simulink library "custom_blocks"  (R2019b)
settings: Solver=VariableStepAuto  StartTime=0.0  StopTime=10.0  RelTol=1e-3
undefined symbols (not defined in the file): aMode, National_Instruments, PCIe, samp
libraries: simulink x25, powerlib_meascontrol x9, $bdroot x2, sldrtlib x1
(part 1 of 2)
settings Model: Creator=guy-m  LastModifiedBy=guy-m

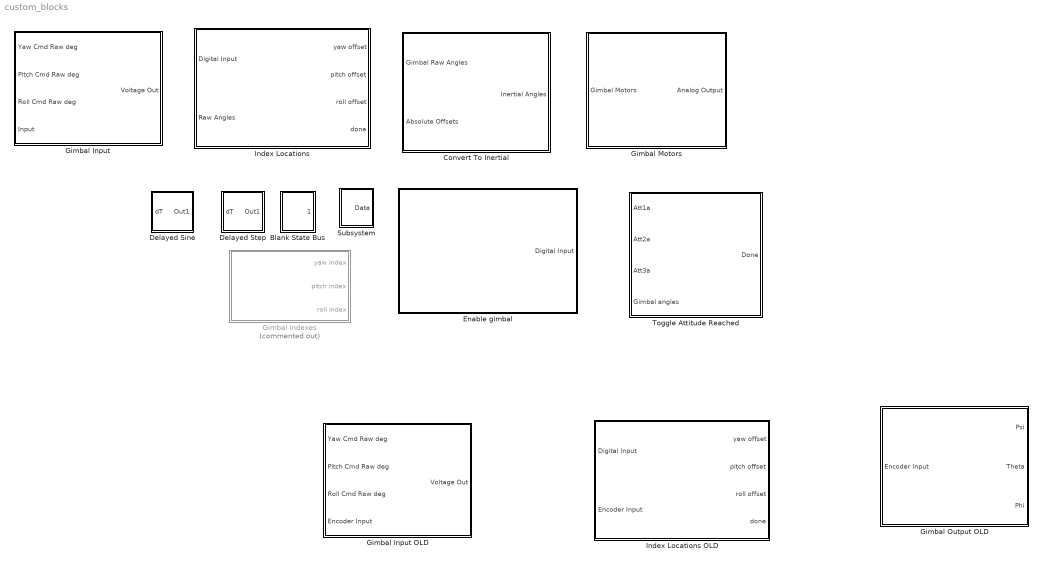
== system custom_blocks ==
  Blank State Bus : Subsystem
      mask DialogControl DescTextVar Prompt: Just a sample state bus object
      mask Display: disp("Blank\nState\nBus")
  Convert To Inertial : Subsystem
      mask init:
      | requiredBlock = find_system(bdroot,'name','Enable gimbal');
      | yawOffset = str2num(get_param(requiredBlock{1},'yawOffset'));
      | pitchOffset = str2num(get_param(requiredBlock{1},'pitchOffset'));
      | rollOffset = str2num(get_param(requiredBlock{1},'rollOffset'));
      mask Display:
      | text(0.5,1," Raw 2 Inertial \n (degrees)",'verticalAlignment','top',"horizontalAlignment",'center')
      | port_label('output',1,'Inertial Angles','texmode','on');
      | port_label('input',1,'Raw Output','texmode','on');
      | port_label('input',2,'Abs. Offsets','texmode','on');
  Delayed Sine : Subsystem  mask{amp=1, bias=5, freq=pi, phase=pi, onTime=0, duration=inf}
      mask DialogControl Control2 Prompt: Amplitude:
      mask DialogControl Control3 Prompt: Bias:
      mask DialogControl Control4 Prompt: Frequency (rad/s):
      mask DialogControl Control5 Prompt: Phase (rad):
      mask DialogControl Control6_copy Prompt: Relative On-Time (s)
      mask DialogControl Control6 Prompt: Duration (s)
      mask Display:
      | port_label('output',1,'','texmode','off');
      | port_label('input',1,'dt','texmode','on');
      | 
      | x = 0:0.001:1;
      | y = sin(2*pi*x);
      | 
      | x = [0,(x+0.5)];
      | y = [0,y];
      | 
      | plot(x,y)
  Delayed Step : Subsystem  mask{stepTime=1, u0=5, u1=pi}
      mask help: This block is similar to a step input, except that the step time is delayed by the block input value (in seconds)
      mask DialogControl Control2 Prompt: Step time:
      mask DialogControl Control3 Prompt: Initial value:
      mask DialogControl Control4 Prompt: Final value:
      mask Display:
      | port_label('output',1,'','texmode','off');
      | port_label('input',1,'dt','texmode','on');
      | if u1>=u0
      |     x = [0.1 0.5 0.5 0.9];
      |     y = [0.1 0.1 0.9 0.9];
      | else
      |     x = [0.1 0.5 0.5 0.9];
      |     y = [0.9 0.9 0.1 0.1];
      | end
      | 
      | plot(x,y)
  Enable gimbal : Subsystem  mask{yawOffset=0, pitchOffset=0, rollOffset=0}
      mask DialogControl DescTextVar Prompt: This block is required in order to enable interfacing with the flight table
      mask DialogControl Control2 Prompt: Yaw Euler Offset
      mask DialogControl Control3 Prompt: Pitch Euler Offset
      mask DialogControl Control4 Prompt: Roll Euler Offset
      mask Display:
      | text(0.5,1,"Enable Gimbals",'verticalAlignment','top',"horizontalAlignment",'center')
      | 
      | port_label('output',1,'Digital Input','texmode','on');
  Gimbal Indexes : Subsystem  Commented=on
      mask Display:
      | disp("Detect Change\nGimbal Index")
      | port_label('output',1,'Yaw','texmode','on');
      | port_label('output',2,'Pitch','texmode','on');
      | port_label('output',3,'Roll','texmode','on');
  Gimbal Input : Subsystem
      mask init: same as custom_blocks/Convert To Inertial
      mask DialogControl DescTextVar Prompt: This block send the raw attitude angles to the gimbal
      mask Display:
      | disp("Gimbal Input\n(degrees)");
      | port_label('input',1,'Yaw','texmode','on');
      | port_label('input',2,'Pitch','texmode','on');
      | port_label('input',3,'Roll','texmode','on');
      | port_label('input',4,'Input','texmode','on');
      | port_label('output',1,'Motors','texmode','on');
  Gimbal Input OLD : Subsystem
      mask init: same as custom_blocks/Convert To Inertial
      mask DialogControl DescTextVar Prompt: This block send the raw attitude angles to the gimbal
      mask Display:
      | disp("Gimbal Input\n(degrees)");
      | port_label('input',1,'Yaw','texmode','on');
      | port_label('input',2,'Pitch','texmode','on');
      | port_label('input',3,'Roll','texmode','on');
      | port_label('input',4,'Encoder Input','texmode','on');
      | port_label('output',1,'Motors','texmode','on');
  Gimbal Motors : Subsystem
      mask DialogControl DescTextVar Prompt: This block controls the DC motors of the gimbal
      mask DialogControl DescTextVar_copy Prompt: A bus object with voltages for each yaw, pitch, and roll motors
      mask Display:
      | text(0.5,1,"Gimbal Motors",'verticalAlignment','top',"horizontalAlignment",'center')
      | 
      | port_label('output',1,"Analog Output",'texmode','on');
      | port_label('input',1,"Motor Voltages",'texmode','on');
  Gimbal Output OLD : Subsystem
      mask init: same as custom_blocks/Convert To Inertial
      mask Display:
      | text(0.5,1," Gimbal Attitude\n (degrees)",'verticalAlignment','top',"horizontalAlignment",'center')
      | port_label('output',1,'Yaw','texmode','on');
      | port_label('output',2,'Pitch','texmode','on');
      | port_label('output',3,'Roll','texmode','on');
      | port_label('input',1,'Encoder Input','texmode','on');
  Index Locations : Subsystem
      mask init: same as custom_blocks/Convert To Inertial
      mask DialogControl DescTextVar Prompt: This block sends (relative) angles at which the physical indexes are found
      mask Display:
      | disp("Gimbal Indexes\n(degrees)")
      | port_label('output',1,'Yaw','texmode','on');
      | port_label('output',2,'Pitch','texmode','on');
      | port_label('output',3,'Roll','texmode','on');
      | port_label('output',4,'Done','texmode','on');
      | port_label('input',1,'Digital Input','texmode','on');
      | port_label('input',2,'Raw Output','texmode','on');
  Index Locations OLD : Subsystem
      mask DialogControl DescTextVar Prompt: This block sends (relative) angles at which the physical indexes are found
      mask Display:
      | disp("Gimbal Indexes\n(degrees)")
      | port_label('output',1,'Yaw','texmode','on');
      | port_label('output',2,'Pitch','texmode','on');
      | port_label('output',3,'Roll','texmode','on');
      | port_label('output',4,'Done','texmode','on');
      | port_label('input',1,'Digital Input','texmode','on');
      | port_label('input',2,'Encoder Input','texmode','on');
  Subsystem : Subsystem
      mask DialogControl ParameterGroupVar Prompt: Just a sample Pixhawk serial message
      mask Display: disp("Blank\nPixhawk\nInput")
  Toggle Attitude Reached : Subsystem
      mask DialogControl DescTextVar Prompt: This block outputs 'true' as soon as both sets of attitude angles coinside. This is a one-time toggle! once turned on, it will remain this way forever.
      mask Display:
      | disp("Toggle Attitude Reached")
      | 
      | port_label('input',1,'Yaw_1','texmode','on');
      | port_label('input',2,'Pitch_1','texmode','on');
      | port_label('input',3,'Roll_1','texmode','on');
      | port_label('input',4,'Encoder Input','texmode','on');
      | port_label('output',1,'Toggle','texmode','on');

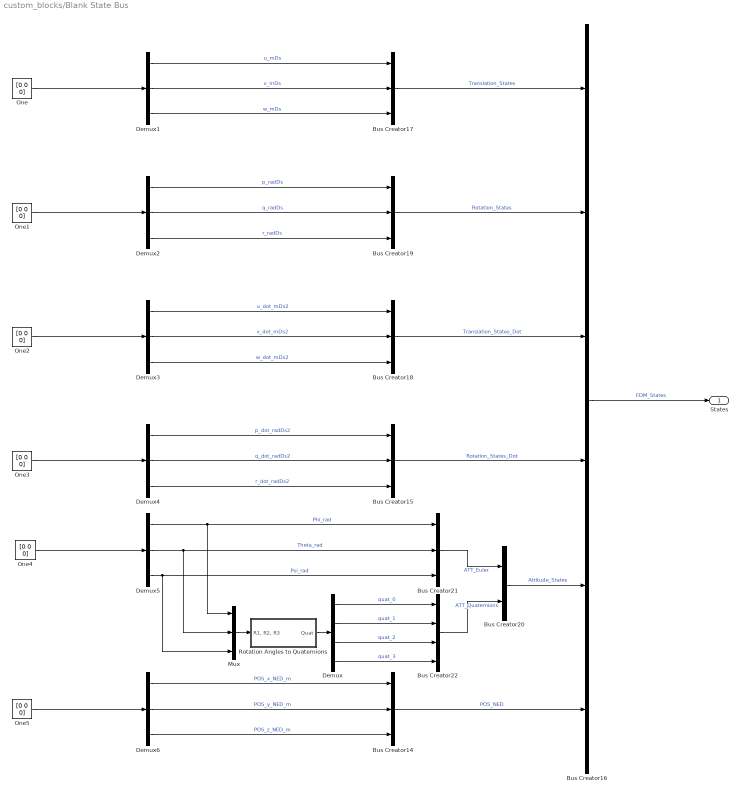
== system custom_blocks/Blank State Bus ==
  Bus Creator{14..15,17..19,21} (6 alike) : BusCreator  Inputs=3
  Bus Creator16 : BusCreator  Inputs=6
  Bus Creator20 : BusCreator  Inputs=2
  Bus Creator22 : BusCreator  Inputs=4
  Demux : Demux
  Demux{1..6} (6 alike) : Demux  Outputs=3
  Mux : Mux  Inputs=3
  One{,1..5} (6 alike) : Constant  Value=[0 0 0]  OutDataTypeStr=Inherit: Inherit via back propagation
  Rotation Angles to Quaternions : Subsystem  mask(Ang2Quat){rotationOrder=ZYX, aMode=aMode}
      mask prompts: rotationOrder "shared_aeroblks:sharedaeroblktransform:blockAng2QuatParamRotationOrder"
      mask help: shared_aeroblks:sharedaeroblktransform:blockAng2QuatDesc
      mask init:
      | if aerosharedtest(gcb)
      |     ports=aerosharedicon('sharedang2quat');
      | else
      |     ports=sharedautoicon('sharedang2quat');
      | end
      settings: AttributesFormatString=Rotation Order: %<rotationOrder>
      mask Help: eval('if license(''test'',''Aerospace_Blockset'')aerosharedhelp(''rotation_angles_to_quaternions'');elseif license(''test'',''Powertrain_Blockset'')sharedautohelp(''rotation_angles_to_quaternions'');end')
      mask TypeOptions rotationOrder: shared_aeroblks:sharedaeroblktransform:blockParamComboZYX | shared_aeroblks:sharedaeroblktransform:blockParamComboZYZ | shared_aeroblks:sharedaeroblktransform:blockParamComboZXY | shared_aeroblks:sharedaeroblktransform:blockParamComboZXZ | shared_aeroblks:sharedaeroblktransform:blockParamComboYXZ | shared_aeroblks:sharedaeroblktransform:blockParamComboYXY | shared_aeroblks:sharedaeroblktransform:blockParamComboYZX | shared_aeroblks:sharedaeroblktransform:blockParamComboYZY | shared_aeroblks:sharedaeroblktransform:blockParamComboXYZ | shared_aeroblks:sharedaeroblktransform:blockParamComboXYX | shared_aeroblks:sharedaeroblktransform:blockParamComboXZY | shared_aeroblks:sharedaeroblktransform:blockParamComboXZX
      mask DialogControl rotationOrder Prompt: Rotation order:
      mask Display:
      | port_label('input',1,'[R_1,R_2,R_3]','texmode','on')
      | port_label('output',1,'q','texmode','on')
  "States " : Outport  VectorParamsAs1DForOutWhenUnconnected=off
  wires:
  One2/1 -> Demux3/1
  Bus Creator22/1 -> Bus Creator20/2  "ATT_Quaternions"
  Bus Creator15/1 -> Bus Creator16/4  "Rotation_States_Dot"
  Demux4/1 -> Bus Creator15/1  "p_dot_radDs2"
  Bus Creator14/1 -> Bus Creator16/6  "POS_NED"
  Demux/3 -> Bus Creator22/3  "quat_2"
  Bus Creator16/1 -> "States "/1  "FDM_States"
  Rotation Angles to Quaternions/1(Quat) -> Demux/1
  Demux/2 -> Bus Creator22/2  "quat_1"
  Demux/4 -> Bus Creator22/4  "quat_3"
  Demux2/2 -> Bus Creator19/2  "q_radDs"
  Mux/1 -> Rotation Angles to Quaternions/1("R1, R2, R3")
  Bus Creator18/1 -> Bus Creator16/3  "Translation_States_Dot"
  Bus Creator17/1 -> Bus Creator16/1  "Translation_States"
  Demux6/1 -> Bus Creator14/1  "POS_x_NED_m"
  Bus Creator21/1 -> Bus Creator20/1  "ATT_Euler"
  Demux6/3 -> Bus Creator14/3  "POS_z_NED_m"
  Bus Creator20/1 -> Bus Creator16/5  "Attitude_States"
  Demux5/2 -> Mux/2, Bus Creator21/2  "Theta_rad"
  Demux5/3 -> Mux/3, Bus Creator21/3  "Psi_rad"
  One1/1 -> Demux2/1
  Demux3/2 -> Bus Creator18/2  "v_dot_mDs2"
  Demux1/2 -> Bus Creator17/2  "v_mDs"
  Demux4/3 -> Bus Creator15/3  "r_dot_radDs2"
  Bus Creator19/1 -> Bus Creator16/2  "Rotation_States"
  Demux2/3 -> Bus Creator19/3  "r_radDs"
  Demux1/1 -> Bus Creator17/1  "u_mDs"
  Demux2/1 -> Bus Creator19/1  "p_radDs"
  Demux3/3 -> Bus Creator18/3  "w_dot_mDs2"
  Demux/1 -> Bus Creator22/1  "quat_0"
  Demux5/1 -> Mux/1, Bus Creator21/1  "Phi_rad"
  Demux1/3 -> Bus Creator17/3  "w_mDs"
  Demux4/2 -> Bus Creator15/2  "q_dot_radDs2"
  Demux6/2 -> Bus Creator14/2  "POS_y_NED_m"
  Demux3/1 -> Bus Creator18/1  "u_dot_mDs2"
  One3/1 -> Demux4/1
  One4/1 -> Demux5/1
  One/1 -> Demux1/1
  One5/1 -> Demux6/1

== system custom_blocks/Convert To Inertial ==
  Gimbal Raw Angles : Inport
  Absolute Offsets : Inport  Port=2
  Bus Creator : BusCreator  Inputs=3
  Bus Selector : BusSelector  OutputSignals=yawAbsOffset,pitchAbsOffset,rollAbsOffset
  Bus Selector1 : BusSelector  OutputSignals=yawRaw,pitchRaw,rollRaw
  Constant : Constant  Value=yawOffset
  Constant1 : Constant  Value=pitchOffset
  Constant2 : Constant  Value=rollOffset
  Subtract : Sum  Inputs=+++
  Subtract1 : Sum  Inputs=+++
  Subtract2 : Sum  Inputs=+++
  Inertial Angles : Outport
  wires:
  Bus Selector/3 -> Subtract2/3  "<rollAbsOffset>"
  Bus Selector/2 -> Subtract1/3  "<pitchAbsOffset>"
  Bus Selector/1 -> Subtract/3  "<yawAbsOffset>"
  Absolute Offsets/1 -> Bus Selector/1
  Constant2/1 -> Subtract2/1
  Constant1/1 -> Subtract1/1
  Constant/1 -> Subtract/1
  Subtract2/1 -> Bus Creator/3  "inertialRoll"
  Subtract1/1 -> Bus Creator/2  "inertialPitch"
  Subtract/1 -> Bus Creator/1  "inertialYaw"
  Bus Selector1/2 -> Subtract1/2  "<pitchRaw>"
  Bus Selector1/1 -> Subtract/2  "<yawRaw>"
  Bus Selector1/3 -> Subtract2/2  "<rollRaw>"
  Gimbal Raw Angles/1 -> Bus Selector1/1
  Bus Creator/1 -> Inertial Angles/1

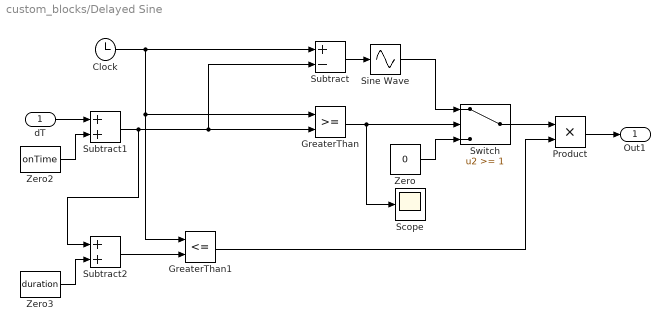
== system custom_blocks/Delayed Sine ==
  dT : Inport
  Clock : Clock
  GreaterThan : RelationalOperator  OutDataTypeStr=boolean  RndMeth=Simplest
  GreaterThan1 : RelationalOperator  Operator=<=  OutDataTypeStr=boolean  RndMeth=Simplest
  Product : Product
  Scope : Scope
  Sine Wave : Sin  TimeSource=Use external signal  Amplitude=amp  Bias=bias  Frequency=freq  Phase=phase  SampleTime=samp
  Subtract : Sum  Inputs=+-
  Subtract1 : Sum
  Subtract2 : Sum
  Switch : Switch  Threshold=1
  Zero : Constant  Value=0  OutDataTypeStr=Inherit: Inherit via back propagation
  Zero2 : Constant  Value=onTime  OutDataTypeStr=Inherit: Inherit via back propagation
  Zero3 : Constant  Value=duration  OutDataTypeStr=Inherit: Inherit via back propagation
  Out1 : Outport
  wires:
  Clock/1 -> GreaterThan1/1, GreaterThan/1, Subtract/1
  GreaterThan/1 -> Switch/2, Scope/1
  Sine Wave/1 -> Switch/1
  Switch/1 -> Product/1
  Zero/1 -> Switch/3
  Subtract/1 -> Sine Wave/1
  Subtract1/1 -> Subtract2/1, GreaterThan/2, Subtract/2
  Product/1 -> Out1/1
  GreaterThan1/1 -> Product/2
  dT/1 -> Subtract1/1
  Zero2/1 -> Subtract1/2
  Zero3/1 -> Subtract2/2
  Subtract2/1 -> GreaterThan1/2

== system custom_blocks/Delayed Step ==
  dT : Inport
  Clock : Clock
  Constant1 : Constant  Value=u0
  Constant2 : Constant  Value=stepTime
  Constant3 : Constant  Value=u1
  GreaterThan : RelationalOperator  OutDataTypeStr=boolean  RndMeth=Simplest
  Scope : Scope
  Sum : Sum
  Switch : Switch  Threshold=1
  Out1 : Outport
  wires:
  Switch/1 -> Out1/1
  Constant1/1 -> Switch/3
  Constant3/1 -> Switch/1
  GreaterThan/1 -> Switch/2, Scope/1
  dT/1 -> Sum/1
  Clock/1 -> GreaterThan/1
  Sum/1 -> GreaterThan/2
  Constant2/1 -> Sum/2

== system custom_blocks/Enable gimbal ==
  Mux digCont : Mux  Inputs=2
  enable : Constant  SampleTime=-1
  stop : Constant  Value=0  SampleTime=-1
  Digital Input : Outport
  wires:
  stop/1 -> Mux digCont/2
  Mux digCont/1 -> Digital Input/1
  enable/1 -> Mux digCont/1

== system custom_blocks/Gimbal Indexes ==
  note: This block sends a pulse each time a gimbal axis crosses the hardware index
  note: short delay to avoid reading false positive at 0 seconds
  Clock : Clock
  Compare To Constant : simulink/Logic and Bit Operations/Compare To Constant  relop=>=  const=0.005  OutDataTypeStr=boolean
  Demux2 : Demux  Outputs=3
  Digital Input1 : sldrtlib/Digital Input  SampleTime=0.001  MaxMissedTicks=100  ShowMissedTicks=off  YieldWhenWaiting=off  DrvName=National_Instruments/PCIe-6353  DrvAddress=4294967295  DrvOptions=[0 15 0 2 2 2 2]  Channels=[45:47]  BitMode=1  DataType=1
      settings: AttributesFormatString=National Instruments\nPCIe-6353 [auto]  SourceProductName=Simulink Desktop Real-Time  SourceProductBaseCode=WT
  Edge Detector : powerlib_meascontrol/Logic/Edge Detector  model=Either  ic=0  Ts=0
      settings: SourceProductName=Simscape Electrical  SourceProductBaseCode=PS
  Edge Detector1 : powerlib_meascontrol/Logic/Edge Detector  model=Either  ic=0  Ts=0
      settings: SourceProductName=Simscape Electrical  SourceProductBaseCode=PS
  Edge Detector2 : powerlib_meascontrol/Logic/Edge Detector  model=Either  ic=0  Ts=0
      settings: SourceProductName=Simscape Electrical  SourceProductBaseCode=PS
  Product : Product
  Product1 : Product
  Product2 : Product
  yaw index : Outport  InitialOutput=0
  pitch index : Outport  Port=2  InitialOutput=0
  roll index : Outport  Port=3  InitialOutput=0
  wires:
  Digital Input1/1 -> Demux2/1
  Demux2/1 -> Edge Detector/1
  Demux2/2 -> Edge Detector1/1
  Demux2/3 -> Edge Detector2/1
  Edge Detector/1 -> Product/2
  Edge Detector1/1 -> Product1/2
  Edge Detector2/1 -> Product2/2
  Clock/1 -> Compare To Constant/1
  Product/1 -> yaw index/1
  Product1/1 -> pitch index/1
  Product2/1 -> roll index/1
  Compare To Constant/1 -> Product2/1, Product1/1, Product/1

== system custom_blocks/Gimbal Input ==
  note: Old Controllers
  Yaw Cmd Raw deg : Inport
  Pitch Cmd Raw deg : Inport  Port=2
  Roll Cmd Raw deg : Inport  Port=3
  Input : Inport  Port=4
  Bus Creator : BusCreator  Inputs=3
  Demux : Demux  Outputs=3
  PITCH : Subsystem
  PITCH1 : Subsystem  Commented=on
  ROLL : Subsystem
  ROLL1 : Subsystem  Commented=on
  YAW : Subsystem
  YAW1 : Subsystem  Commented=on
  Voltage Out : Outport
  wires:
  ROLL/1(Phi Motor Voltage) -> Bus Creator/3  "phi voltage"
  YAW/1(Psi Motor Voltage) -> Bus Creator/1  "psi voltage"
  Demux/1 -> YAW/2(Psi Meas)  "yaw"
  Demux/2 -> PITCH/2(Theta Meas)  "pitch"
  Demux/3 -> ROLL/2(Phi Meas)  "roll"
  PITCH/1(Theta Motor Voltage) -> Bus Creator/2  "theta voltage"
  Bus Creator/1 -> Voltage Out/1
  Yaw Cmd Raw deg/1 -> YAW/1(Psi Cmd)
  Pitch Cmd Raw deg/1 -> PITCH/1(Theta Cmd)
  Roll Cmd Raw deg/1 -> ROLL/1(Phi Cmd)
  Input/1 -> Demux/1

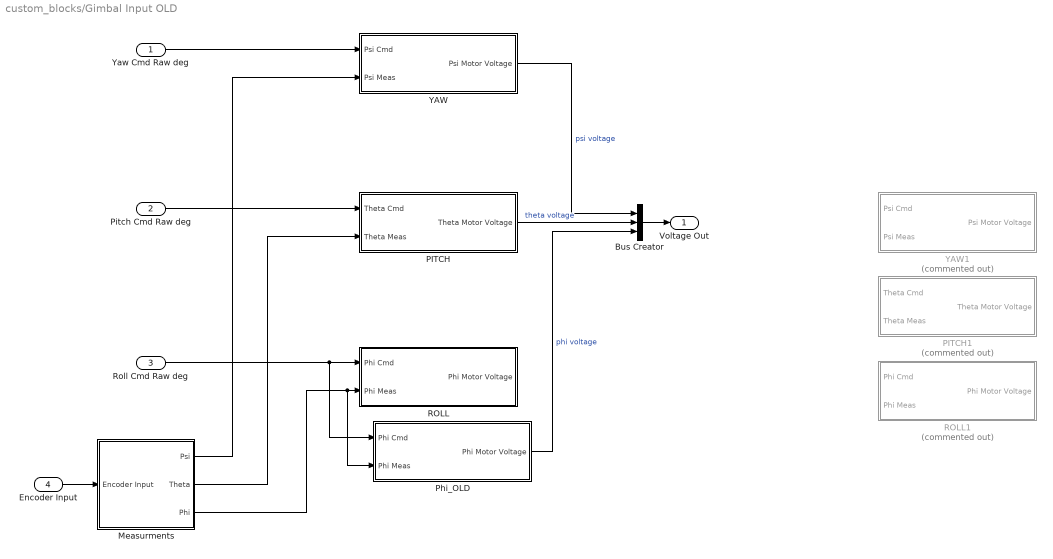
== system custom_blocks/Gimbal Input OLD ==
  Yaw Cmd Raw deg : Inport
  Pitch Cmd Raw deg : Inport  Port=2
  Roll Cmd Raw deg : Inport  Port=3
  Encoder Input : Inport  Port=4
  Bus Creator : BusCreator  Inputs=3
  Measurments : Subsystem
  PITCH : Subsystem
  PITCH1 : Subsystem  Commented=on  AncestorBlock=custom_blocks/Gimbal Input/PITCH
  "Phi_OLD " : Subsystem
  ROLL : Subsystem
  ROLL1 : Subsystem  Commented=on  AncestorBlock=custom_blocks/Gimbal Input/ROLL
  YAW : Subsystem
  YAW1 : Subsystem  Commented=on  AncestorBlock=custom_blocks/Gimbal Input/YAW
  Voltage Out : Outport
  wires:
  Encoder Input/1 -> Measurments/1(Encoder Input)
  Roll Cmd Raw deg/1 -> ROLL/1(Phi Cmd), "Phi_OLD "/1(Phi Cmd)
  Pitch Cmd Raw deg/1 -> PITCH/1(Theta Cmd)
  Yaw Cmd Raw deg/1 -> YAW/1(Psi Cmd)
  Bus Creator/1 -> Voltage Out/1
  PITCH/1(Theta Motor Voltage) -> Bus Creator/2  "theta voltage"
  Measurments/3(Phi) -> ROLL/2(Phi Meas), "Phi_OLD "/2(Phi Meas)
  Measurments/2(Theta) -> PITCH/2(Theta Meas)
  Measurments/1(Psi) -> YAW/2(Psi Meas)
  YAW/1(Psi Motor Voltage) -> Bus Creator/1  "psi voltage"
  "Phi_OLD "/1(Phi Motor Voltage) -> Bus Creator/3  "phi voltage"

== system custom_blocks/Gimbal Motors ==
  Gimbal Motors : Inport
  Bus Creator : BusCreator  Commented=on  Inputs=3
  Bus Selector : BusSelector  OutputSignals=psi voltage,theta voltage,phi voltage
  Phi deadzone : Subsystem
  Subsystem : Subsystem
  Subsystem1 : Subsystem
  Zero : Constant  Commented=on  Value=0  OutDataTypeStr=Inherit: Inherit via back propagation
  Zero1 : Constant  Commented=on  Value=0  OutDataTypeStr=Inherit: Inherit via back propagation
  Zero2 : Constant  Commented=on  Value=0  OutDataTypeStr=Inherit: Inherit via back propagation
  control Mux : Mux  Inputs=3
  Analog Output : Outport
  wires:
  Bus Selector/2 -> Subsystem/1(Theta U)  "<theta voltage>"
  Bus Selector/1 -> Subsystem1/1(Psi U)  "<psi voltage>"
  control Mux/1 -> Analog Output/1
  Gimbal Motors/1 -> Bus Selector/1
  Bus Selector/3 -> Phi deadzone/1(Phi U)  "<phi voltage>"
  Phi deadzone/1(Phi V) -> control Mux/3
  Subsystem/1(Theta V) -> control Mux/2
  Subsystem1/1(Psi V) -> control Mux/1
  Zero/1 -> Bus Creator/1  "psi voltage"
  Zero1/1 -> Bus Creator/2  "theta voltage"
  Zero2/1 -> Bus Creator/3  "phi voltage"

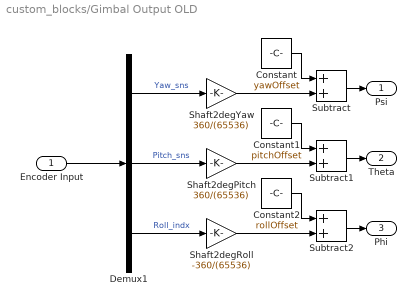
== system custom_blocks/Gimbal Output OLD ==
  Encoder Input : Inport
  Constant : Constant  Value=yawOffset
  Constant1 : Constant  Value=pitchOffset
  Constant2 : Constant  Value=rollOffset
  Demux1 : Demux  Outputs=3
  Shaft2degPitch : Gain  Gain=360/(65536)
  Shaft2degRoll : Gain  Gain=-360/(65536)
  Shaft2degYaw : Gain  Gain=360/(65536)
  Subtract : Sum
  Subtract1 : Sum
  Subtract2 : Sum
  Psi : Outport
  Theta : Outport  Port=2
  Phi : Outport  Port=3
  wires:
  Encoder Input/1 -> Demux1/1
  Demux1/3 -> Shaft2degRoll/1  "Roll_indx"
  Shaft2degRoll/1 -> Subtract2/2
  Demux1/2 -> Shaft2degPitch/1  "Pitch_sns"
  Demux1/1 -> Shaft2degYaw/1  "Yaw_sns"
  Shaft2degYaw/1 -> Subtract/2
  Shaft2degPitch/1 -> Subtract1/2
  Subtract/1 -> Psi/1
  Subtract1/1 -> Theta/1
  Subtract2/1 -> Phi/1
  Constant/1 -> Subtract/1
  Constant1/1 -> Subtract1/1
  Constant2/1 -> Subtract2/1

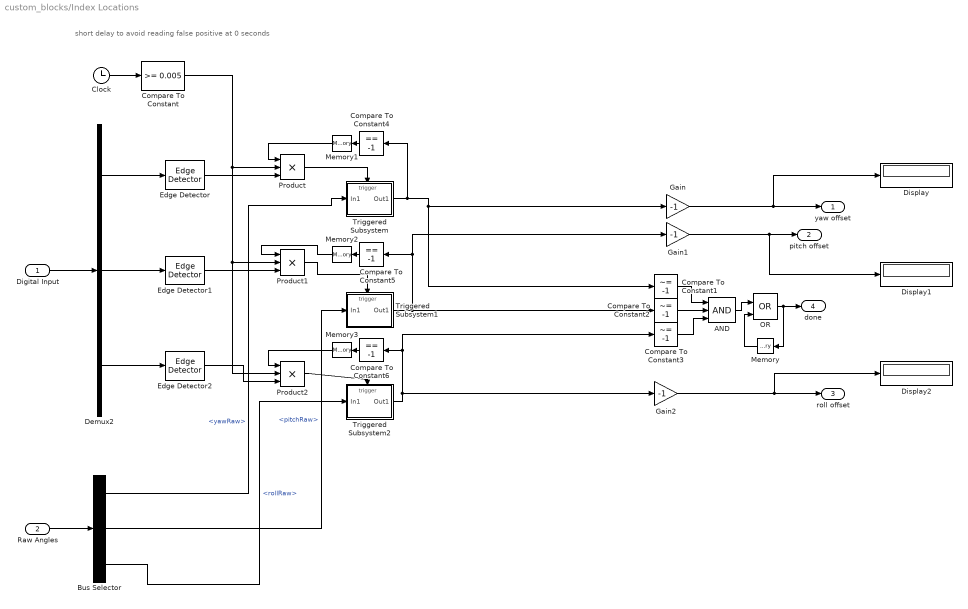
== system custom_blocks/Index Locations ==
  note: short delay to avoid reading false positive at 0 seconds
  Digital Input : Inport
  Raw Angles : Inport  Port=2
  AND : Logic  Inputs=3  IconShape=distinctive  AllPortsSameDT=off  OutDataTypeStr=boolean
  Bus Selector : BusSelector  OutputSignals=yawRaw,pitchRaw,rollRaw
  Clock : Clock
  Compare To Constant : simulink/Logic and Bit Operations/Compare To Constant  relop=>=  const=0.005  OutDataTypeStr=boolean
  Compare To Constant1 : simulink/Logic and Bit Operations/Compare To Constant  relop=~=  const=-1  OutDataTypeStr=boolean
  Compare To Constant2 : simulink/Logic and Bit Operations/Compare To Constant  relop=~=  const=-1  OutDataTypeStr=boolean
  Compare To Constant3 : simulink/Logic and Bit Operations/Compare To Constant  relop=~=  const=-1  OutDataTypeStr=boolean
  Compare To Constant4 : simulink/Logic and Bit Operations/Compare To Constant  relop===  const=-1  OutDataTypeStr=boolean
  Compare To Constant5 : simulink/Logic and Bit Operations/Compare To Constant  relop===  const=-1  OutDataTypeStr=boolean
  Compare To Constant6 : simulink/Logic and Bit Operations/Compare To Constant  relop===  const=-1  OutDataTypeStr=boolean
  Demux2 : Demux  Outputs=3
  Display : Display
  Display1 : Display
  Display2 : Display
  Edge Detector : powerlib_meascontrol/Logic/Edge Detector  model=Either  ic=0  Ts=0
      settings: SourceProductName=Simscape Electrical  SourceProductBaseCode=PS
  Edge Detector1 : powerlib_meascontrol/Logic/Edge Detector  model=Either  ic=0  Ts=0
      settings: SourceProductName=Simscape Electrical  SourceProductBaseCode=PS
  Edge Detector2 : powerlib_meascontrol/Logic/Edge Detector  model=Either  ic=0  Ts=0
      settings: SourceProductName=Simscape Electrical  SourceProductBaseCode=PS
  Gain : Gain  Gain=-1
  Gain1 : Gain  Gain=-1
  Gain2 : Gain  Gain=-1
  Memory{,1..3} (4 alike) : Memory
  OR : Logic  Operator=OR  IconShape=distinctive  AllPortsSameDT=off  OutDataTypeStr=boolean
  Product : Product  Inputs=3
  Product1 : Product  Inputs=3
  Product2 : Product  Inputs=3
  Triggered Subsystem : Subsystem  TreatAsAtomicUnit=on
  Triggered Subsystem1 : Subsystem  TreatAsAtomicUnit=on
  Triggered Subsystem2 : Subsystem  TreatAsAtomicUnit=on
  yaw offset : Outport  InitialOutput=0
  pitch offset : Outport  Port=2  InitialOutput=0
  roll offset : Outport  Port=3  InitialOutput=0
  done : Outport  Port=4  InitialOutput=0
  wires:
  Triggered Subsystem2/1(Out1) -> Compare To Constant3/1, Compare To Constant6/1, Gain2/1
  Triggered Subsystem1/1(Out1) -> Gain1/1, Compare To Constant5/1, Compare To Constant2/1
  Triggered Subsystem/1(Out1) -> Gain/1, Compare To Constant1/1, Compare To Constant4/1
  Raw Angles/1 -> Bus Selector/1
  Memory/1 -> OR/2
  OR/1 -> done/1, Memory/1
  AND/1 -> OR/1
  Compare To Constant3/1 -> AND/3
  Compare To Constant2/1 -> AND/2
  Compare To Constant1/1 -> AND/1
  Product2/1 -> Triggered Subsystem2/Trigger
  Bus Selector/3 -> Triggered Subsystem2/1(In1)  "<rollRaw>"
  Product1/1 -> Triggered Subsystem1/Trigger
  Bus Selector/2 -> Triggered Subsystem1/1(In1)  "<pitchRaw>"
  Bus Selector/1 -> Triggered Subsystem/1(In1)  "<yawRaw>"
  Product/1 -> Triggered Subsystem/Trigger
  Compare To Constant/1 -> Product2/2, Product1/2, Product/2
  Digital Input/1 -> Demux2/1
  Demux2/2 -> Edge Detector1/1
  Demux2/1 -> Edge Detector/1
  Demux2/3 -> Edge Detector2/1
  Clock/1 -> Compare To Constant/1
  Edge Detector/1 -> Product/3
  Edge Detector2/1 -> Product2/3
  Edge Detector1/1 -> Product1/3
  Memory1/1 -> Product/1
  Compare To Constant4/1 -> Memory1/1
  Compare To Constant5/1 -> Memory2/1
  Memory2/1 -> Product1/1
  Compare To Constant6/1 -> Memory3/1
  Memory3/1 -> Product2/1
  Gain/1 -> yaw offset/1, Display/1
  Gain1/1 -> Display1/1, pitch offset/1
  Gain2/1 -> roll offset/1, Display2/1

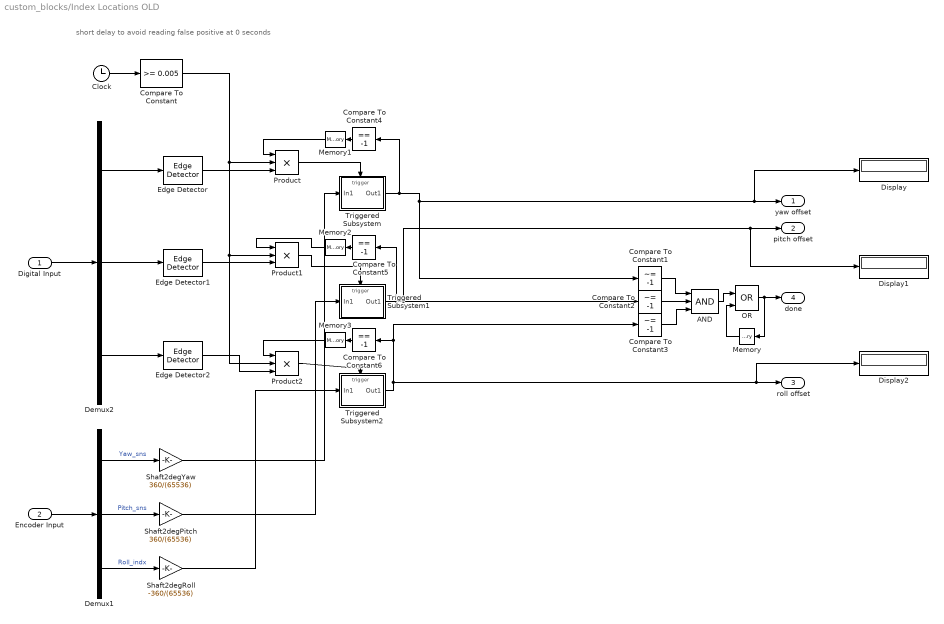
== system custom_blocks/Index Locations OLD ==
  note: short delay to avoid reading false positive at 0 seconds
  Digital Input : Inport
  Encoder Input : Inport  Port=2
  AND : Logic  Inputs=3  IconShape=distinctive  AllPortsSameDT=off  OutDataTypeStr=boolean
  Clock : Clock
  Compare To Constant : simulink/Logic and Bit Operations/Compare To Constant  relop=>=  const=0.005  OutDataTypeStr=boolean
  Compare To Constant1 : simulink/Logic and Bit Operations/Compare To Constant  relop=~=  const=-1  OutDataTypeStr=boolean
  Compare To Constant2 : simulink/Logic and Bit Operations/Compare To Constant  relop=~=  const=-1  OutDataTypeStr=boolean
  Compare To Constant3 : simulink/Logic and Bit Operations/Compare To Constant  relop=~=  const=-1  OutDataTypeStr=boolean
  Compare To Constant4 : simulink/Logic and Bit Operations/Compare To Constant  relop===  const=-1  OutDataTypeStr=boolean
  Compare To Constant5 : simulink/Logic and Bit Operations/Compare To Constant  relop===  const=-1  OutDataTypeStr=boolean
  Compare To Constant6 : simulink/Logic and Bit Operations/Compare To Constant  relop===  const=-1  OutDataTypeStr=boolean
  Demux1 : Demux  Outputs=3
  Demux2 : Demux  Outputs=3
  Display : Display
  Display1 : Display
  Display2 : Display
  Edge Detector : powerlib_meascontrol/Logic/Edge Detector  model=Either  ic=0  Ts=0
      settings: SourceProductName=Simscape Electrical  SourceProductBaseCode=PS
  Edge Detector1 : powerlib_meascontrol/Logic/Edge Detector  model=Either  ic=0  Ts=0
      settings: SourceProductName=Simscape Electrical  SourceProductBaseCode=PS
  Edge Detector2 : powerlib_meascontrol/Logic/Edge Detector  model=Either  ic=0  Ts=0
      settings: SourceProductName=Simscape Electrical  SourceProductBaseCode=PS
  Memory{,1..3} (4 alike) : Memory
  OR : Logic  Operator=OR  IconShape=distinctive  AllPortsSameDT=off  OutDataTypeStr=boolean
  Product : Product  Inputs=3
  Product1 : Product  Inputs=3
  Product2 : Product  Inputs=3
  Shaft2degPitch : Gain  Gain=360/(65536)
  Shaft2degRoll : Gain  Gain=-360/(65536)
  Shaft2degYaw : Gain  Gain=360/(65536)
  Triggered Subsystem : Subsystem  TreatAsAtomicUnit=on
  Triggered Subsystem1 : Subsystem  TreatAsAtomicUnit=on
  Triggered Subsystem2 : Subsystem  TreatAsAtomicUnit=on
  yaw offset : Outport  InitialOutput=0
  pitch offset : Outport  Port=2  InitialOutput=0
  roll offset : Outport  Port=3  InitialOutput=0
  done : Outport  Port=4  InitialOutput=0
  wires:
  Memory3/1 -> Product2/1
  Compare To Constant6/1 -> Memory3/1
  Memory2/1 -> Product1/1
  Compare To Constant5/1 -> Memory2/1
  Compare To Constant4/1 -> Memory1/1
  Memory1/1 -> Product/1
  Demux1/2 -> Shaft2degPitch/1  "Pitch_sns"
  Demux1/1 -> Shaft2degYaw/1  "Yaw_sns"
  Demux1/3 -> Shaft2degRoll/1  "Roll_indx"
  Encoder Input/1 -> Demux1/1
  Edge Detector1/1 -> Product1/3
  Edge Detector2/1 -> Product2/3
  Edge Detector/1 -> Product/3
  Clock/1 -> Compare To Constant/1
  Demux2/3 -> Edge Detector2/1
  Demux2/1 -> Edge Detector/1
  Demux2/2 -> Edge Detector1/1
  Digital Input/1 -> Demux2/1
  Compare To Constant/1 -> Product/2, Product1/2, Product2/2
  Product/1 -> Triggered Subsystem/Trigger
  Triggered Subsystem/1(Out1) -> Compare To Constant4/1, Compare To Constant1/1, yaw offset/1, Display/1
  Shaft2degYaw/1 -> Triggered Subsystem/1(In1)
  Shaft2degPitch/1 -> Triggered Subsystem1/1(In1)
  Triggered Subsystem1/1(Out1) -> pitch offset/1, Display1/1, Compare To Constant2/1, Compare To Constant5/1
  Product1/1 -> Triggered Subsystem1/Trigger
  Shaft2degRoll/1 -> Triggered Subsystem2/1(In1)
  Triggered Subsystem2/1(Out1) -> roll offset/1, Display2/1, Compare To Constant6/1, Compare To Constant3/1
  Product2/1 -> Triggered Subsystem2/Trigger
  Compare To Constant1/1 -> AND/1
  Compare To Constant2/1 -> AND/2
  Compare To Constant3/1 -> AND/3
  AND/1 -> OR/1
  OR/1 -> Memory/1, done/1
  Memory/1 -> OR/2

== system custom_blocks/Subsystem ==
  Cast To Double2 : DataTypeConversion  OutDataTypeStr=single
  Constant : Constant  Value=[0 0 0 0 0 0 0 0 0 0 0]  OutDataTypeStr=single
  Heartbeat : simulink/Sources/Counter Free-Running  NumBits=16  tsamp=-1
  Mux : Mux  Inputs=2
  Data : Outport
  wires:
  Cast To Double2/1 -> Mux/1  "send"
  Mux/1 -> Data/1
  Heartbeat/1 -> Cast To Double2/1
  Constant/1 -> Mux/2  "send"

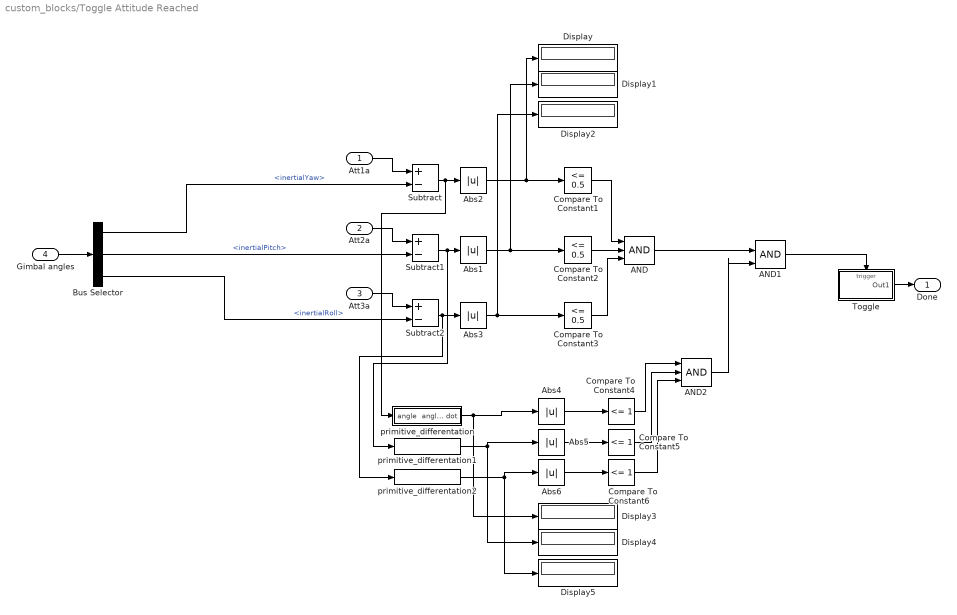
== system custom_blocks/Toggle Attitude Reached ==
  Att1a : Inport
  Att2a : Inport  Port=2
  Att3a : Inport  Port=3
  Gimbal angles : Inport  Port=4
  AND : Logic  Inputs=3  IconShape=distinctive  AllPortsSameDT=off  OutDataTypeStr=boolean
  AND1 : Logic  IconShape=distinctive  AllPortsSameDT=off  OutDataTypeStr=boolean
  AND2 : Logic  Inputs=3  IconShape=distinctive  AllPortsSameDT=off  OutDataTypeStr=boolean
  Abs{1..6} (6 alike) : Abs
  Bus Selector : BusSelector  OutputSignals=inertialYaw,inertialPitch,inertialRoll
  Compare To Constant1 : simulink/Logic and Bit Operations/Compare To Constant  relop=<=  const=0.5  OutDataTypeStr=boolean
  Compare To Constant2 : simulink/Logic and Bit Operations/Compare To Constant  relop=<=  const=0.5  OutDataTypeStr=boolean
  Compare To Constant3 : simulink/Logic and Bit Operations/Compare To Constant  relop=<=  const=0.5  OutDataTypeStr=boolean
  Compare To Constant4 : simulink/Logic and Bit Operations/Compare To Constant  relop=<=  const=1  OutDataTypeStr=boolean
  Compare To Constant5 : simulink/Logic and Bit Operations/Compare To Constant  relop=<=  const=1  OutDataTypeStr=boolean
  Compare To Constant6 : simulink/Logic and Bit Operations/Compare To Constant  relop=<=  const=1  OutDataTypeStr=boolean
  Display{,1..5} (6 alike) : Display
  Subtract : Sum  Inputs=+-
  Subtract1 : Sum  Inputs=+-
  Subtract2 : Sum  Inputs=+-
  Toggle : Subsystem  TreatAsAtomicUnit=on
  primitive_differentation : Subsystem
  primitive_differentation1 : $bdroot/Toggle Attitude Reached/primitive_differentation  SystemSampleTime=-1  Latency=0  AutoFrameSizeCalculation=off
  primitive_differentation2 : $bdroot/Toggle Attitude Reached/primitive_differentation  SystemSampleTime=-1  Latency=0  AutoFrameSizeCalculation=off
  Done : Outport
  wires:
  Abs3/1 -> Compare To Constant3/1, Display2/1
  Abs1/1 -> Compare To Constant2/1, Display1/1
  Abs2/1 -> Compare To Constant1/1, Display/1
  Toggle/1(Out1) -> Done/1
  Att3a/1 -> Subtract2/1
  Att2a/1 -> Subtract1/1
  AND/1 -> AND1/1
  Compare To Constant1/1 -> AND/1
  Compare To Constant3/1 -> AND/3
  Att1a/1 -> Subtract/1
  Compare To Constant2/1 -> AND/2
  Subtract/1 -> primitive_differentation/1(angle), Abs2/1
  Subtract1/1 -> primitive_differentation1/1, Abs1/1
  Subtract2/1 -> primitive_differentation2/1, Abs3/1
  primitive_differentation/1(angle dot) -> Display3/1, Abs4/1
  primitive_differentation1/1 -> Display4/1, Abs5/1
  primitive_differentation2/1 -> Display5/1, Abs6/1
  Compare To Constant4/1 -> AND2/1
  Compare To Constant5/1 -> AND2/2
  Compare To Constant6/1 -> AND2/3
  AND2/1 -> AND1/2
  AND1/1 -> Toggle/Trigger
  Abs4/1 -> Compare To Constant4/1
  Abs5/1 -> Compare To Constant5/1
  Abs6/1 -> Compare To Constant6/1
  Bus Selector/1 -> Subtract/2  "<inertialYaw>"
  Bus Selector/2 -> Subtract1/2  "<inertialPitch>"
  Bus Selector/3 -> Subtract2/2  "<inertialRoll>"
  Gimbal angles/1 -> Bus Selector/1

== system custom_blocks/Blank State Bus/Rotation Angles to Quaternions ==
  "R1, R2, R3" : Inport  Unit=rad
  1/2 : Gain  Gain=0.5  SaturateOnIntegerOverflow=on  OutDataTypeStr=Inherit: Same as input  ParamDataTypeStr=Inherit: Same as input
  Mux1 : Mux  Inputs=2
  Mux2 : Mux
  q0 : Fcn  Expr=u(4)*u(5)*u(6) + u(1)*u(2)*u(3)
  q1 : Fcn  Expr=u(4)*u(5)*u(3) - u(1)*u(2)*u(6)
  q2 : Fcn  Expr=u(4)*u(2)*u(6) + u(1)*u(5)*u(3)
  q3 : Fcn  Expr=u(1)*u(5)*u(6) - u(4)*u(2)*u(3)
  sincos : Trigonometry  Operator=sincos
  Quat : Outport  Unit=1  InitialOutput=0  VectorParamsAs1DForOutWhenUnconnected=off
  wires:
  q0/1 -> Mux2/1
  Mux2/1 -> Quat/1
  q3/1 -> Mux2/4
  q2/1 -> Mux2/3
  q1/1 -> Mux2/2
  Mux1/1 -> q3/1, q2/1, q1/1, q0/1
  sincos/2 -> Mux1/2
  sincos/1 -> Mux1/1
  1/2/1 -> sincos/1
  "R1, R2, R3"/1 -> 1/2/1

== system custom_blocks/Gimbal Input/PITCH ==
  Theta Cmd : Inport
  Theta Meas : Inport  Port=2
  Cin : Gain  Gain=0.05
  Cout : DiscreteTransferFcn  Numerator="[24600      -23400]"  Denominator="[ 1                      -0.6]"
  Diff with Low Pass : DiscreteTransferFcn  Numerator="[95.2380952380952         -95.2380952380952]"  Denominator="[1        -0.904761904761905]"
  Low Pass : DiscreteTransferFcn  Numerator="[0.111111111111111         0.111111111111111]"  Denominator="[1        -0.777777777777778]"
  Saturation2 : Saturate  UpperLimit=150  LowerLimit=-150
  Sum : Sum  Inputs=|+-
  Sum1 : Sum  Inputs=|+-
  error1 : Scope
  Theta Motor Voltage : Outport
  wires:
  Sum/1 -> Cout/1
  Diff with Low Pass/1 -> error1/1, Sum1/2  "Phi dot"
  Cin/1 -> Low Pass/1
  Cout/1 -> Saturation2/1
  Sum1/1 -> Cin/1
  Saturation2/1 -> Sum1/1
  Theta Cmd/1 -> Sum/1
  Theta Meas/1 -> Diff with Low Pass/1, Sum/2
  Low Pass/1 -> Theta Motor Voltage/1  "Phi dot"

== system custom_blocks/Gimbal Input/PITCH1 ==
  Theta Cmd : Inport
  Theta Meas : Inport  Port=2
  Cin1 : TransferFcn  Numerator="[0.60923                   30.4615]"  Denominator=[1 200]
  Constant1 : Constant  Value=180
  Gain : Gain
  Manual Switch1 : ManualSwitch
  Saturation1 : Saturate  UpperLimit=180  LowerLimit=-180
  Sum : Sum  Inputs=|+-
  Sum1 : Sum  Inputs=|+-
  Transfer Fcn1 : TransferFcn  Numerator=[1 0]  Denominator=[0.01 1]
  Transfer Fcn3 : TransferFcn  Numerator=|  Denominator=|
      Numerator=|
      | [1280.01863570108 238830.820154417 11694377.8192853
      | ]
      Denominator=|
      | [1 313.302916162976 53156.2628149332
      | ]
  Theta Motor Voltage : Outport
  wires:
  Sum1/1 -> Cin1/1
  Gain/1 -> Transfer Fcn3/1
  Transfer Fcn3/1 -> Saturation1/1
  Sum/1 -> Gain/1
  Transfer Fcn1/1 -> Sum1/2
  Theta Cmd/1 -> Manual Switch1/1
  Constant1/1 -> Manual Switch1/2
  Cin1/1 -> Theta Motor Voltage/1
  Theta Meas/1 -> Sum/2, Transfer Fcn1/1
  Saturation1/1 -> Sum1/1
  Manual Switch1/1 -> Sum/1

== system custom_blocks/Gimbal Input/ROLL ==
  Phi Cmd : Inport
  Phi Meas : Inport  Port=2
  Cin : Gain  Gain=0.025
  Cout : DiscreteTransferFcn  Numerator=|  Denominator="[1                      -0.6]"
      | [   820  -780
      | ]
  Diff with Low Pass : DiscreteTransferFcn  Numerator="[95.2380952380952         -95.2380952380952]"  Denominator="[1        -0.904761904761905]"
  Saturation2 : Saturate  UpperLimit=350  LowerLimit=-350
  Sum : Sum  Inputs=|+-
  Sum1 : Sum  Inputs=|+-
  error1 : Scope
  Phi Motor Voltage : Outport
  wires:
  Sum/1 -> Cout/1
  Diff with Low Pass/1 -> error1/1, Sum1/2  "Phi dot"
  Cin/1 -> Phi Motor Voltage/1
  Cout/1 -> Saturation2/1
  Sum1/1 -> Cin/1
  Saturation2/1 -> Sum1/1
  Phi Cmd/1 -> Sum/1
  Phi Meas/1 -> Diff with Low Pass/1, Sum/2

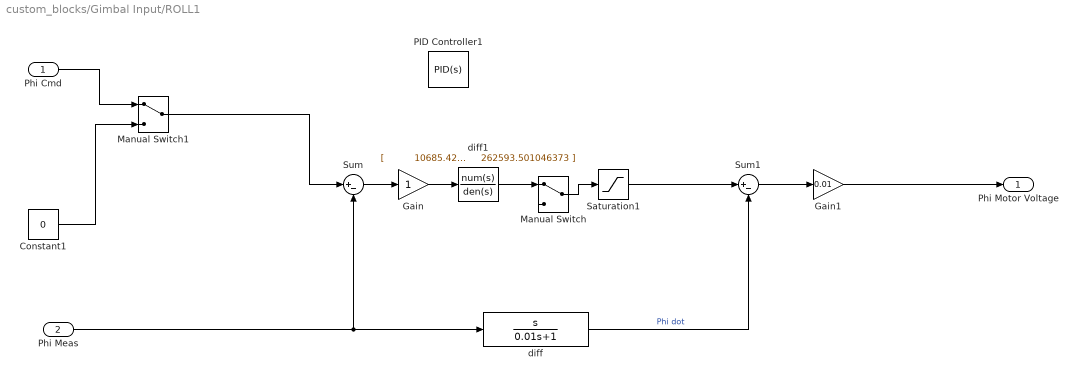
== system custom_blocks/Gimbal Input/ROLL1 ==
  Phi Cmd : Inport
  Phi Meas : Inport  Port=2
  Constant1 : Constant  Value=0
  Gain : Gain
  Gain1 : Gain  Gain=0.01
  Manual Switch : ManualSwitch
  Manual Switch1 : ManualSwitch
  PID Controller1 : simulink/Continuous/PID Controller  Controller=PID  Form=Parallel  TimeDomain=Continuous-time  SampleTime=-1  IntegratorMethod=Forward Euler  FilterMethod=Forward Euler  ControllerParametersSource=internal  P=20  I=0  D=0  UseFilter=on  N=100  TunerSelectOption=Transfer Function Based (PID Tuner App)  InitialConditionSource=internal  InitialConditionForIntegrator=0  InitialConditionForFilter=0  DifferentiatorICPrevScaledInput=0  ExternalReset=none  TrackingMode=off  Kt=1  LimitOutput=off  UpperSaturationLimit=inf  LowerSaturationLimit=-inf  LinearizeAsGain=on  AntiWindupMode=none  Kb=1  POutMin=[]  POutMax=[]  IOutMin=[]  IOutMax=[]  DOutMin=[]  DOutMax=[]  NOutMin=[]  NOutMax=[]  SumOutMin=[]  SumOutMax=[]  SaturationOutMin=[]  SaturationOutMax=[]  PParamMin=[]  PParamMax=[]  IParamMin=[]  IParamMax=[]  DParamMin=[]  DParamMax=[]  NParamMin=[]  NParamMax=[]  KbParamMin=[]  KbParamMax=[]  KtParamMin=[]  KtParamMax=[]  KbOutMin=[]  KbOutMax=[]  KtOutMin=[]  KtOutMax=[]  IntegratorOutMin=[]  IntegratorOutMax=[]  FilterOutMin=[]  FilterOutMax=[]  SumI1OutMin=[]  SumI1OutMax=[]  SumI2OutMin=[]  SumI2OutMax=[]  SumI3OutMin=[]  SumI3OutMax=[]  SumI4OutMin=[]  SumI4OutMax=[]  SumDOutMin=[]  SumDOutMax=[]  DifferentiatorOutMin=[]  DifferentiatorOutMax=[]  FilterDiffOutCoefMin=[]  FilterDiffOutCoefMax=[]  ReciprocalOutMin=[]  ReciprocalOutMax=[]  SumDenOutMin=[]  SumDenOutMax=[]  SumNumOutMin=[]  SumNumOutMax=[]  DivideOutMin=[]  DivideOutMax=[]  IntegratorContinuousStateAttributes=''  IntegratorStateMustResolveToSignalObject=off  IntegratorRTWStateStorageClass=Auto  FilterContinuousStateAttributes=''  FilterStateMustResolveToSignalObject=off  FilterRTWStateStorageClass=Auto  ParallelPVariant=InternalParameters  IdealPVariant=Disabled  IVariant=InternalParameters  DVariant=InternalParameters  IntegratorVariant=Continuous  SatVariant=Disabled  AWVariant=Passthrough  PCopyVariant=Disabled  TRVariant=Disabled  FdbkBlocksVariant=Forward  IdealPFdbkVariant=Disabled  SatFdbkVariant=Disabled  DerivativeFilterVariant=ContFilter  NVariant=InternalParameters  NCopyVariant=Disabled  FilterICVariant=InternalICsFilter  IntegratorICVariant=InternalICs  ExternalResetVariant=Disabled  TRSumVariant=Passthrough  SumFdbkVariant=Disabled  SumVariant=Sum_PID
  Saturation1 : Saturate  UpperLimit=300  LowerLimit=-300
  Sum : Sum  Inputs=|+-
  Sum1 : Sum  Inputs=|+-
  diff : TransferFcn  Numerator=[1 0]  Denominator=[0.01 1]
  diff1 : TransferFcn  Numerator=|  Denominator=|
      Numerator=|
      | [          10685.4236488389          2993753.33796508          236334150.941735
      | ]
      Denominator=|
      | [                         1          1020.23062031815          262593.501046373
      | ]
  Phi Motor Voltage : Outport
  wires:
  Sum/1 -> Gain/1
  Manual Switch/1 -> Saturation1/1
  diff1/1 -> Manual Switch/1
  diff/1 -> Sum1/2  "Phi dot"
  Phi Meas/1 -> Sum/2, diff/1
  Sum1/1 -> Gain1/1
  Saturation1/1 -> Sum1/1
  Manual Switch1/1 -> Sum/1
  Constant1/1 -> Manual Switch1/2
  Phi Cmd/1 -> Manual Switch1/1
  Gain/1 -> diff1/1
  Gain1/1 -> Phi Motor Voltage/1

== system custom_blocks/Gimbal Input/YAW ==
  Psi Cmd : Inport
  Psi Meas : Inport  Port=2
  Cin : Gain  Gain=0.08
  Cout : DiscreteTransferFcn  Numerator="[ 13038.4615384615         -12602.5641025641]"  Denominator=|
      | [1        -0.709401709401709
      | ]
  Diff with Low Pass : DiscreteTransferFcn  Numerator="[95.2380952380952         -95.2380952380952]"  Denominator="[1        -0.904761904761905]"
  Low Pass : DiscreteTransferFcn  Commented=through  Numerator="[0.0769230769230769        0.0769230769230769]"  Denominator="[1        -0.846153846153846]"
  Saturation2 : Saturate  UpperLimit=100  LowerLimit=-100
  Sum : Sum  Inputs=|+-
  Sum1 : Sum  Inputs=|+-
  error1 : Scope
  Psi Motor Voltage : Outport
  wires:
  Diff with Low Pass/1 -> error1/1, Sum1/2  "Phi dot"
  Psi Meas/1 -> Diff with Low Pass/1, Sum/2
  Saturation2/1 -> Sum1/1
  Psi Cmd/1 -> Sum/1
  Sum/1 -> Cout/1
  Cout/1 -> Saturation2/1
  Cin/1 -> Low Pass/1
  Sum1/1 -> Cin/1
  Low Pass/1 -> Psi Motor Voltage/1  "Phi dot"

== system custom_blocks/Gimbal Input/YAW1 ==
  Psi Cmd : Inport
  Psi Meas : Inport  Port=2
  Cin : TransferFcn  Numerator=2.9192*[1 53.87]  Denominator=[1 200]
  Constant1 : Constant  Value=180
  Gain : Gain
  Manual Switch1 : ManualSwitch
  Saturation2 : Saturate  UpperLimit=100  LowerLimit=-100
  Sum : Sum  Inputs=|+-
  Sum1 : Sum  Inputs=|+-
  Transfer Fcn1 : TransferFcn  Numerator=|  Denominator=|
      Numerator=|
      | [          1048.88683783117          153388.518090953          10291300.4472415
      | ]
      Denominator=|
      | [                         1          457.625701221523           57405.478732949
      | ]
  Zero-Order Hold3 : ZeroOrderHold  SampleTime=0.01
  diff : TransferFcn  Numerator=[1 0]  Denominator=[0.01 1]
  error1 : Scope
  Psi Motor Voltage : Outport
  wires:
  Sum1/1 -> Cin/1
  Gain/1 -> Transfer Fcn1/1
  Zero-Order Hold3/1 -> Psi Motor Voltage/1
  Cin/1 -> Zero-Order Hold3/1  "Phi"
  Transfer Fcn1/1 -> Saturation2/1
  Sum/1 -> Gain/1
  Constant1/1 -> Manual Switch1/2
  Psi Cmd/1 -> Manual Switch1/1
  Manual Switch1/1 -> Sum/1
  Saturation2/1 -> Sum1/1
  Psi Meas/1 -> Sum/2, diff/1
  diff/1 -> Sum1/2, error1/1  "Phi dot"

== system custom_blocks/Gimbal Input OLD/Measurments ==
  Encoder Input : Inport
  Constant : Constant  Value=yawOffset
  Constant1 : Constant  Value=pitchOffset
  Constant2 : Constant  Value=rollOffset
  Demux1 : Demux  Outputs=3
  Shaft2degPitch : Gain  Gain=360/(65536)
  Shaft2degRoll : Gain  Gain=-360/(65536)
  Shaft2degYaw : Gain  Gain=360/(65536)
  Subtract : Sum
  Subtract1 : Sum
  Subtract2 : Sum
  Psi : Outport
  Theta : Outport  Port=2
  Phi : Outport  Port=3
  wires:
  Constant2/1 -> Subtract2/1
  Constant1/1 -> Subtract1/1
  Constant/1 -> Subtract/1
  Subtract2/1 -> Phi/1
  Subtract1/1 -> Theta/1
  Subtract/1 -> Psi/1
  Shaft2degPitch/1 -> Subtract1/2
  Shaft2degYaw/1 -> Subtract/2
  Demux1/1 -> Shaft2degYaw/1  "Yaw_sns"
  Demux1/2 -> Shaft2degPitch/1  "Pitch_sns"
  Shaft2degRoll/1 -> Subtract2/2
  Demux1/3 -> Shaft2degRoll/1  "Roll_indx"
  Encoder Input/1 -> Demux1/1

== system custom_blocks/Gimbal Input OLD/PITCH ==
  Theta Cmd : Inport
  Theta Meas : Inport  Port=2
  Cin1 : TransferFcn  Numerator="[0.60923                   30.4615]"  Denominator=[1 200]
  Constant1 : Constant  Value=180
  Gain : Gain  Gain=0.1
  Manual Switch1 : ManualSwitch
  Saturation1 : Saturate  UpperLimit=180  LowerLimit=-180
  Sum : Sum  Inputs=|+-
  Sum1 : Sum  Inputs=|+-
  Transfer Fcn1 : TransferFcn  Numerator=[1 0]  Denominator=[0.01 1]
  Transfer Fcn3 : TransferFcn  Numerator=|  Denominator=|
      Numerator=|
      | [1280.01863570108 238830.820154417 11694377.8192853
      | ]
      Denominator=|
      | [1 313.302916162976 53156.2628149332
      | ]
  Theta Motor Voltage : Outport
  wires:
  Sum1/1 -> Cin1/1
  Gain/1 -> Transfer Fcn3/1
  Transfer Fcn3/1 -> Saturation1/1
  Sum/1 -> Gain/1
  Transfer Fcn1/1 -> Sum1/2
  Theta Cmd/1 -> Manual Switch1/1
  Constant1/1 -> Manual Switch1/2
  Cin1/1 -> Theta Motor Voltage/1
  Theta Meas/1 -> Sum/2, Transfer Fcn1/1
  Saturation1/1 -> Sum1/1
  Manual Switch1/1 -> Sum/1

== system custom_blocks/Gimbal Input OLD/PITCH1 ==
  Theta Cmd : Inport
  Theta Meas : Inport  Port=2
  Cin1 : TransferFcn  Numerator="[0.60923                   30.4615]"  Denominator=[1 200]
  Constant1 : Constant  Value=180
  Gain : Gain  Gain=0.1
  Manual Switch1 : ManualSwitch
  Saturation1 : Saturate  UpperLimit=180  LowerLimit=-180
  Sum : Sum  Inputs=|+-
  Sum1 : Sum  Inputs=|+-
  Transfer Fcn1 : TransferFcn  Numerator=[1 0]  Denominator=[0.01 1]
  Transfer Fcn3 : TransferFcn  Numerator=|  Denominator=|
      Numerator=|
      | [1280.01863570108 238830.820154417 11694377.8192853
      | ]
      Denominator=|
      | [1 313.302916162976 53156.2628149332
      | ]
  Theta Motor Voltage : Outport
  wires:
  Manual Switch1/1 -> Sum/1
  Saturation1/1 -> Sum1/1
  Theta Meas/1 -> Transfer Fcn1/1, Sum/2
  Cin1/1 -> Theta Motor Voltage/1
  Constant1/1 -> Manual Switch1/2
  Theta Cmd/1 -> Manual Switch1/1
  Transfer Fcn1/1 -> Sum1/2
  Sum/1 -> Gain/1
  Transfer Fcn3/1 -> Saturation1/1
  Gain/1 -> Transfer Fcn3/1
  Sum1/1 -> Cin1/1

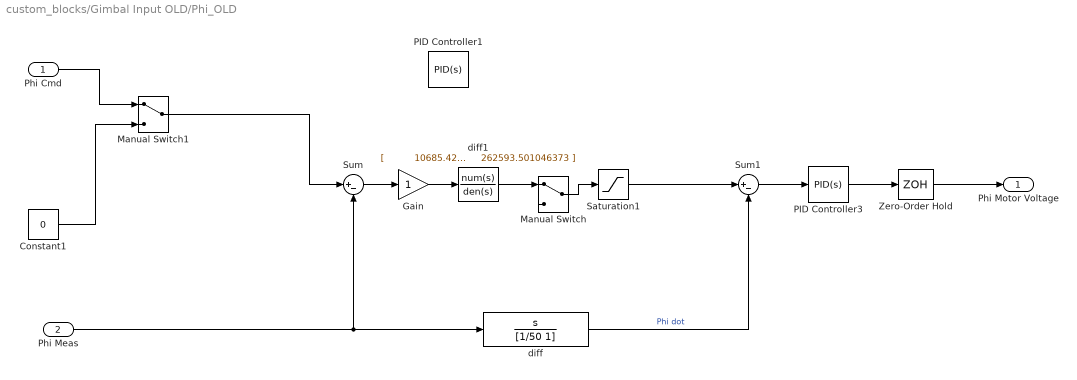
== system custom_blocks/Gimbal Input OLD/Phi_OLD  ==
  Phi Cmd : Inport
  Phi Meas : Inport  Port=2
  Constant1 : Constant  Value=0
  Gain : Gain
  Manual Switch : ManualSwitch
  Manual Switch1 : ManualSwitch
  PID Controller1 : simulink/Continuous/PID Controller  Controller=PID  Form=Parallel  TimeDomain=Continuous-time  SampleTime=-1  IntegratorMethod=Forward Euler  FilterMethod=Forward Euler  ControllerParametersSource=internal  P=20  I=0  D=0  UseFilter=on  N=100  TunerSelectOption=Transfer Function Based (PID Tuner App)  InitialConditionSource=internal  InitialConditionForIntegrator=0  InitialConditionForFilter=0  DifferentiatorICPrevScaledInput=0  ExternalReset=none  TrackingMode=off  Kt=1  LimitOutput=off  UpperSaturationLimit=inf  LowerSaturationLimit=-inf  LinearizeAsGain=on  AntiWindupMode=none  Kb=1  POutMin=[]  POutMax=[]  IOutMin=[]  IOutMax=[]  DOutMin=[]  DOutMax=[]  NOutMin=[]  NOutMax=[]  SumOutMin=[]  SumOutMax=[]  SaturationOutMin=[]  SaturationOutMax=[]  PParamMin=[]  PParamMax=[]  IParamMin=[]  IParamMax=[]  DParamMin=[]  DParamMax=[]  NParamMin=[]  NParamMax=[]  KbParamMin=[]  KbParamMax=[]  KtParamMin=[]  KtParamMax=[]  KbOutMin=[]  KbOutMax=[]  KtOutMin=[]  KtOutMax=[]  IntegratorOutMin=[]  IntegratorOutMax=[]  FilterOutMin=[]  FilterOutMax=[]  SumI1OutMin=[]  SumI1OutMax=[]  SumI2OutMin=[]  SumI2OutMax=[]  SumI3OutMin=[]  SumI3OutMax=[]  SumI4OutMin=[]  SumI4OutMax=[]  SumDOutMin=[]  SumDOutMax=[]  DifferentiatorOutMin=[]  DifferentiatorOutMax=[]  FilterDiffOutCoefMin=[]  FilterDiffOutCoefMax=[]  ReciprocalOutMin=[]  ReciprocalOutMax=[]  SumDenOutMin=[]  SumDenOutMax=[]  SumNumOutMin=[]  SumNumOutMax=[]  DivideOutMin=[]  DivideOutMax=[]  IntegratorContinuousStateAttributes=''  IntegratorStateMustResolveToSignalObject=off  IntegratorRTWStateStorageClass=Auto  FilterContinuousStateAttributes=''  FilterStateMustResolveToSignalObject=off  FilterRTWStateStorageClass=Auto  ParallelPVariant=InternalParameters  IdealPVariant=Disabled  IVariant=InternalParameters  DVariant=InternalParameters  IntegratorVariant=Continuous  SatVariant=Disabled  AWVariant=Passthrough  PCopyVariant=Disabled  TRVariant=Disabled  FdbkBlocksVariant=Forward  IdealPFdbkVariant=Disabled  SatFdbkVariant=Disabled  DerivativeFilterVariant=ContFilter  NVariant=InternalParameters  NCopyVariant=Disabled  FilterICVariant=InternalICsFilter  IntegratorICVariant=InternalICs  ExternalResetVariant=Disabled  TRSumVariant=Passthrough  SumFdbkVariant=Disabled  SumVariant=Sum_PID
  PID Controller3 : simulink/Continuous/PID Controller  Controller=PID  Form=Parallel  TimeDomain=Continuous-time  SampleTime=-1  IntegratorMethod=Forward Euler  FilterMethod=Forward Euler  ControllerParametersSource=internal  P=0.07  I=0  D=0  UseFilter=on  N=100  TunerSelectOption=Transfer Function Based (PID Tuner App)  InitialConditionSource=internal  InitialConditionForIntegrator=0  InitialConditionForFilter=0  DifferentiatorICPrevScaledInput=0  ExternalReset=none  TrackingMode=off  Kt=1  LimitOutput=off  UpperSaturationLimit=inf  LowerSaturationLimit=-inf  LinearizeAsGain=on  AntiWindupMode=none  Kb=1  POutMin=[]  POutMax=[]  IOutMin=[]  IOutMax=[]  DOutMin=[]  DOutMax=[]  NOutMin=[]  NOutMax=[]  SumOutMin=[]  SumOutMax=[]  SaturationOutMin=[]  SaturationOutMax=[]  PParamMin=[]  PParamMax=[]  IParamMin=[]  IParamMax=[]  DParamMin=[]  DParamMax=[]  NParamMin=[]  NParamMax=[]  KbParamMin=[]  KbParamMax=[]  KtParamMin=[]  KtParamMax=[]  KbOutMin=[]  KbOutMax=[]  KtOutMin=[]  KtOutMax=[]  IntegratorOutMin=[]  IntegratorOutMax=[]  FilterOutMin=[]  FilterOutMax=[]  SumI1OutMin=[]  SumI1OutMax=[]  SumI2OutMin=[]  SumI2OutMax=[]  SumI3OutMin=[]  SumI3OutMax=[]  SumI4OutMin=[]  SumI4OutMax=[]  SumDOutMin=[]  SumDOutMax=[]  DifferentiatorOutMin=[]  DifferentiatorOutMax=[]  FilterDiffOutCoefMin=[]  FilterDiffOutCoefMax=[]  ReciprocalOutMin=[]  ReciprocalOutMax=[]  SumDenOutMin=[]  SumDenOutMax=[]  SumNumOutMin=[]  SumNumOutMax=[]  DivideOutMin=[]  DivideOutMax=[]  IntegratorContinuousStateAttributes=''  IntegratorStateMustResolveToSignalObject=off  IntegratorRTWStateStorageClass=Auto  FilterContinuousStateAttributes=''  FilterStateMustResolveToSignalObject=off  FilterRTWStateStorageClass=Auto  ParallelPVariant=InternalParameters  IdealPVariant=Disabled  IVariant=InternalParameters  DVariant=InternalParameters  IntegratorVariant=Continuous  SatVariant=Disabled  AWVariant=Passthrough  PCopyVariant=Disabled  TRVariant=Disabled  FdbkBlocksVariant=Forward  IdealPFdbkVariant=Disabled  SatFdbkVariant=Disabled  DerivativeFilterVariant=ContFilter  NVariant=InternalParameters  NCopyVariant=Disabled  FilterICVariant=InternalICsFilter  IntegratorICVariant=InternalICs  ExternalResetVariant=Disabled  TRSumVariant=Passthrough  SumFdbkVariant=Disabled  SumVariant=Sum_PID
  Saturation1 : Saturate  UpperLimit=300  LowerLimit=-300
  Sum : Sum  Inputs=|+-
  Sum1 : Sum  Inputs=|+-
  Zero-Order Hold : ZeroOrderHold  SampleTime=0.01
  diff : TransferFcn  Numerator=[1 0]  Denominator=[1/50 1]
  diff1 : TransferFcn  Numerator=|  Denominator=|
      Numerator=|
      | [          10685.4236488389          2993753.33796508          236334150.941735
      | ]
      Denominator=|
      | [                         1          1020.23062031815          262593.501046373
      | ]
  Phi Motor Voltage : Outport
  wires:
  Sum/1 -> Gain/1
  Manual Switch/1 -> Saturation1/1
  diff1/1 -> Manual Switch/1
  ? -> Manual Switch/2
  diff/1 -> Sum1/2  "Phi dot"
  Phi Meas/1 -> Sum/2, diff/1
  Sum1/1 -> PID Controller3/1
  Saturation1/1 -> Sum1/1
  Manual Switch1/1 -> Sum/1
  PID Controller3/1 -> Zero-Order Hold/1
  Constant1/1 -> Manual Switch1/2
  Phi Cmd/1 -> Manual Switch1/1
  Gain/1 -> diff1/1
  Zero-Order Hold/1 -> Phi Motor Voltage/1
